simulink model "func2_c"  (R2019b)
settings: Solver=VariableStepAuto  StartTime=0.0  StopTime=10.0  RelTol=1e-3  EnableMultiTasking=on
libraries: ModelComposer x2, templatized_input_2_lib x1
settings Model: Creator=abehbood  LastModifiedBy=abehbood
settings DataIOCC: ReturnWorkspaceOutputs=off
settings OptimizationCC: LifeSpan=inf
settings DebuggingCC: SFUnexpectedBacktrackingDiag=warning  SFNoUnconditionalDefaultTransitionDiag=warning  ArithmeticOperatorsInVariantConditions=warning
settings SFSimCC: SimUseLocalCustomCode=off  CustomCodeUndefinedFunction=UseInterfaceOnly
settings RTWCC: RTWUseLocalCustomCode=off
settings CodeAppCC: StateflowObjectComments=on
settings GRTTargetCC: TargetLangStandard=C89/C90 (ANSI)
settings ConfigComp: CovMetricSettings=dw  CovHtmlReporting=on  CovSaveCumulativeToWorkspaceVar=on  CovSaveSingleToWorkspaceVar=on  CovExternalEMLEnable=off

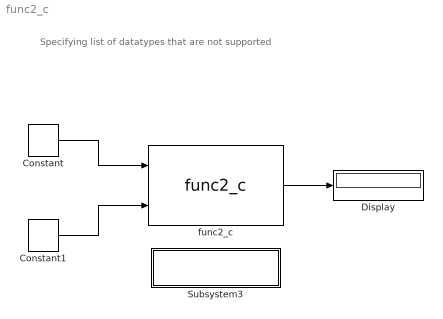
== system func2_c ==
  note: Specifying list of datatypes that are not supported
  Constant : ModelComposer/Constant  Value=40  VectorParams1D=off  SampleTime=1.0  OutDataType=double  TypeExp=''  Signedness=Signed  WordLength=16  FractionalLength=0  RoundingMode=Truncation to minus infinity  OverflowMode=Wrap around
  Constant1 : ModelComposer/Constant  Value=20  VectorParams1D=off  SampleTime=1.0  OutDataType=double  TypeExp=''  Signedness=Signed  WordLength=16  FractionalLength=0  RoundingMode=Truncation to minus infinity  OverflowMode=Wrap around
  Display : Display
  Subsystem3 : Subsystem
      settings: OpenFcn=xmcOpenFileEx
      mask Display: disp(sprintf('Double Click to open\nthe main header file'))
  func2_c : templatized_input_2_lib/func2_c  LibraryFunction=func2_c  IncludeFiles={'func2_c.h'}  SourceFiles={}  IncludeDirectories={}  TemplateParams={'typename T{int8,uint8,int16,uint16,int32,uint32,double,single,half,fixed}'}  FunctionParamTypes={xmcDataType('T'); xmcDataType('T'); xmcDataType('T')}  FunctionParamPassbys={0.000000000000000000e+00; 0.000000000000000000e+00; 0.000000000000000000e+00}  FunctionParamDimensions={'1'; '1'; '1'}  FunctionParamNames={'return'; 'x'; 'y'}  FunctionParamDir={2.000000000000000000e+00; 1.000000000000000000e+00; 1.000000000000000000e+00}  FunctionParamSupportsStreaming={false; false; false}  BufferDepth={'0'}  FunctionParamValues={'0'; '0'; '0'}  ThroughputFactors={''}
  wires:
  Constant/1 -> func2_c/1
  Constant1/1 -> func2_c/2
  func2_c/1 -> Display/1

== system func2_c/Subsystem3 ==
